simulink model "dmpwalk2014"  (R2018b)
settings: Solver=VariableStepAuto  StartTime=0.0  StopTime=100  RelTol=1e-3
values from neighbouring files (symbols this model uses):
  arm_radius = leg_radius    (= 0.01)    [Nao_paramter.m]
  foot_height = 0.02    [Nao_paramter.m]
  foot_length = 0.1    [Nao_paramter.m]
  foot_mass = 0.17184    [Nao_paramter.m]
  foot_width = 0.05    [Nao_paramter.m]
  ground_height = 0.0025    [Nao_paramter.m]
  ground_length = 5    [Nao_paramter.m]
  ground_width = 2    [Nao_paramter.m]
  hand_mass = 0.18533    [Nao_paramter.m]
  head_mass = 0.60533    [Nao_paramter.m]
  hip_mass = 0.14053    [Nao_paramter.m]
  hip_off_Y = 0.05    [Nao_paramter.m]
  hip_off_Z = 0.085    [Nao_paramter.m]
  leg_radius = 0.01    [Nao_paramter.m]
  lowerarm_length = 0.05595    [Nao_paramter.m]
  lowerarm_mass = 0.07761    [Nao_paramter.m]
  neck_length = 0.03    [Nao_paramter.m]
  neck_mass = 0.07842    [Nao_paramter.m]
  neck_off_Z = 0.1265    [Nao_paramter.m]
  shoulder_mass = 0.09304    [Nao_paramter.m]
  thigh_mass = 0.38968    [Nao_paramter.m]
  tibia_mass = 0.30142    [Nao_paramter.m]
  torso_height = foot_height + tibia_length + thigh_length + 0.5*hip_off_Z    (= 0.2654)    [Nao_paramter.m]
  torso_mass = 1.0496    [Nao_paramter.m]
  upperarm_length = 0.105    [Nao_paramter.m]
  upperarm_mass = 0.15777    [Nao_paramter.m]
undefined symbols (not defined in the file or in its folder): sigbuilder_block, X, Y, Z
libraries: sm_lib x87, nesl_utility x15, Contact_Forces_Lib x10
(part 5 of 5)

== stateflow chart dmpwalk2014/motion planning2 ==
  state startStep
    entry:
    tau = 1;
    sDStart = tau*2.04;
    kStartMax = sDStart*100+1;
    [hPil,hPir,kBel,kBer,aPil,aPir,hRol,hRor,aRol,aRor,hYal,hYar] = motionStart(tau);
    state outStart
      entry:
      k = k+1;
      hipRollR = hRor(k);
      hipRollL = hRol(k);
      hipPitchR = hPir(k);
      hipPitchL = hPil(k);
      hipYawR = hYar(k);
      hipYawL = hYal(k);
      kneeBendR = kBer(k);
      kneeBendL = kBel(k);
      ankleRollR = aRor(k);
      ankleRollL = aRol(k);
      anklePitchR = aPir(k);
      anklePitchL = aPil(k);
    (default) -> outStart : {k=0;}
    outStart -> outStart : after(0.01,sec)[k < kStartMax]
  state stepLeft
    entry:
    sDStraight = tau*2.05 ;
    kStraightMax = sDStraight*100+1;
    [hPil,hPir,kBel,kBer,aPil,aPir,hRol,hRor,aRol,aRor,hYal,hYar] = motionStraight(tau,countStraight,motionStartFinal,motionStraightFinal);
    state outLeft
      entry:
      k = k+1;
      hipRollR = hRor(k);
      hipRollL = hRol(k);
      hipPitchR = hPir(k);
      hipPitchL = hPil(k);
      hipYawR = hYar(k);
      hipYawL = hYal(k);
      kneeBendR = kBer(k);
      kneeBendL = kBel(k);
      ankleRollR = aRor(k);
      ankleRollL = aRol(k);
      anklePitchR = aPir(k);
      anklePitchL = aPil(k);
    (default) -> outLeft : {k=0;}
    outLeft -> outLeft : after(0.01,sec)[k < kStraightMax]
  state stepEnd
    entry:
    sDEnd = tau*2.28 ;
    kEndMax = sDEnd*100+1
    [hPil,hPir,kBel,kBer,aPil,aPir,hRol,hRor,aRol,aRor,hYal,hYar] = motionEnd(tau,countEnd,motionStraightFinal,motionEndFinal);
    state outEnd
      entry:
      k = k+1;
      hipRollR = hRor(k);
      hipRollL = hRol(k);
      hipPitchR = hPir(k);
      hipPitchL = hPil(k);
      hipYawR = hYar(k);
      hipYawL = hYal(k);
      kneeBendR = kBer(k);
      kneeBendL = kBel(k);
      ankleRollR = aRor(k);
      ankleRollL = aRol(k);
      anklePitchR = aPir(k);
      anklePitchL = aPil(k);
    (default) -> outEnd : {k=0;}
    outEnd -> outEnd : after(0.01,sec)[k < kEndMax]
  state stepSideR1
    entry:
    sDSideL = tau*2.13;
    kSideLMax = sDSideL*100+1
    [hPil,hPir,kBel,kBer,aPil,aPir,hRol,hRor,aRol,aRor,hYal,hYar] = motionSideLeft(tau,countSide,motionEndFinal,motionSideFinal);
    state outSideR
      entry:
      k = k+1;
      hipRollR = hRor(k);
      hipRollL = hRol(k);
      hipPitchR = hPir(k);
      hipPitchL = hPil(k);
      hipYawR = hYar(k);
      hipYawL = hYal(k);
      kneeBendR = kBer(k);
      kneeBendL = kBel(k);
      ankleRollR = aRor(k);
      ankleRollL = aRol(k);
      anklePitchR = aPir(k);
      anklePitchL = aPil(k);
    (default) -> outSideR : {k=0;}
    outSideR -> outSideR : after(0.01,sec)[k < kSideLMax]
  state stepSideR
    entry:
    sDSideR = tau*2.13;
    kSideRMax = sDSideR*100+1
    [hPil,hPir,kBel,kBer,aPil,aPir,hRol,hRor,aRol,aRor,hYal,hYar] = motionSideRight(tau,countSide,motionEndFinal,motionSideFinal);
    state outSideL
      entry:
      k = k+1;
      hipRollR = hRor(k);
      hipRollL = hRol(k);
      hipPitchR = hPir(k);
      hipPitchL = hPil(k);
      hipYawR = hYar(k);
      hipYawL = hYal(k);
      kneeBendR = kBer(k);
      kneeBendL = kBel(k);
      ankleRollR = aRor(k);
      ankleRollL = aRol(k);
      anklePitchR = aPir(k);
      anklePitchL = aPil(k);
    (default) -> outSideL : {k=0;}
    outSideL -> outSideL : after(0.01,sec)[k < kSideRMax]
  state stepKick
    entry:
    sDKick = tau*2.8 ;
    kKickMax = sDKick*100+1
    [hPil,hPir,kBel,kBer,aPil,aPir,hRol,hRor,aRol,aRor,hYal,hYar] = motionKick(tau,countKick,motionSideFinal,motionKickFinal);
    state outStraight
      entry:
      k = k+1;
      hipRollR = -hRor(k);
      hipRollL = -hRol(k);
      hipPitchR = hPir(k);
      hipPitchL = hPil(k);
      hipYawR = hYar(k);
      hipYawL = hYal(k);
      kneeBendR = kBer(k);
      kneeBendL = kBel(k);
      ankleRollR = -aRor(k);
      ankleRollL = -aRol(k);
      anklePitchR = aPir(k);
      anklePitchL = aPil(k);
    (default) -> outStraight : {k=0;}
    outStraight -> outStraight : after(0.01,sec)[k < kKickMax]
  state stop
    entry:
    stop = 1;
    stopWalking(stop);
    state stopWalking(in) [function]
  (default) -> startStep
  startStep -> stepLeft : after(sDStart,sec){nStraight = 10; countStraight=1;motionStraightFinal = zeros(10,1);motionStraighFinal = zeros(10,1);motionStartFinal = [hPil(k);hPir(k);kBel(k);kBer(k);aPil(k);aPir(k);hRol(k);hRor(k);aRol(k);aRor(k)]; tau = 1;}
  stepLeft -> (junction 880) : after(sDStraight,sec){nStraight = nStraight - 1;motionStraightFinal = [hPil(k);hPir(k);kBel(k);kBer(k);aPil(k);aPir(k);hRol(k);hRor(k);aRol(k);aRor(k)];}
  (junction 880) -> stepEnd [order 2] : [nStraight < 0]{nEnd = 1; countEnd = 1; motionEndFinal = zeros(10,1);tau=1}
  (junction 880) -> stepLeft [order 1] : [nStraight > 0]{countStraight = countStraight+1;}
  stepEnd -> (junction 914) : after(sDEnd,sec){nSide = 20; countSide = 1; motionEndFinal = [hPil(k);hPir(k);kBel(k);kBer(k);aPil(k);aPir(k);hRol(k);hRor(k);aRol(k);aRor(k)]; motionSideFinal = zeros(10,1); LR = 1; tau = 1}
  (junction 914) -> stepSideR1 [order 1] : [LR == 1]
  (junction 914) -> stepSideR [order 2] : [LR == 0]
  (junction 918) -> stepSideR [order 1] : [nSide > 0]{countSide = countSide+1;}
  (junction 918) -> stepSideR1 [order 2] : [nSide > 0]{countSide = countSide+1;}
  stepSideR1 -> (junction 918) : after(sDSideL,sec){nSide = nSide-1;motionSideFinal = [hPil(k);hPir(k);kBel(k);kBer(k);aPil(k);aPir(k);hRol(k);hRor(k);aRol(k);aRor(k)]}
  stepSideR -> (junction 918) : after(sDSideR,sec){nSide = nSide-1;motionSideFinal = [hPil(k);hPir(k);kBel(k);kBer(k);aPil(k);aPir(k);hRol(k);hRor(k);aRol(k);aRor(k)]}
  (junction 918) -> stepKick [order 3] : [after(nSide <= 0,sec]){nKick = 1; countKick = 1; mtionKickFinal = zeros(10,1);}
  (junction 688) -> stepKick [order 1] : [nKick > 0]{countKick = countKick+1;}
  stepKick -> (junction 688) : after(sDKick,sec){nKick = nKick-1; motionKickFinal = [hPil(k);hPir(k);kBel(k);kBer(k);aPil(k);aPir(k);hRol(k);hRor(k);aRol(k);aRor(k)];}
  (junction 688) -> stop [order 2] : [nKick <= 0]
  data: hPl function_output; hPr function_output; kBl function_output; kBr function_output; aPl function_output; aPr function_output; hRl function_output; tScale function_input; hRr function_output; aRl function_output; aRr function_output; hYl function_output; hYr function_output; hPl function_output; hPr function_output; kBl function_output; kBr function_output; aPl function_output; aPr function_output; hRl function_output; tScale function_input; count function_input; hRr function_output; aRl function_output; aRr function_output; hYl function_output; hYr function_output; ygStart function_input; ygStraight function_input; hPl function_output; hPr function_output; kBl function_output; kBr function_output; aPl function_output; aPr function_output; hRl function_output; tScale function_input; count function_input; ygStraight function_input; hRr function_output; aRl function_output; aRr function_output; hYl function_output; hYr function_output; ygEnd function_input; hPl function_output; hPr function_output; kBl function_output; kBr function_output; aPl function_output; aPr function_output; hRl function_output; tScale function_input; count function_input; ygEnd function_input; hRr function_output; aRl function_output; aRr function_output; hYl function_output; hYr function_output; ygSideLeft function_input; hPl function_output; hPr function_output; kBl function_output; kBr function_output; aPl function_output; aPr function_output; hRl function_output; tScale function_input; count function_input; ygEnd function_input; ygSideRight function_input; hRr function_output; aRl function_output; aRr function_output; hYl function_output; hYr function_output; hPl function_output; hPr function_output; kBl function_output; kBr function_output; aPl function_output; aPr function_output; hRl function_output; tScale function_input; count function_input; ygSide function_input; hRr function_output; aRl function_output; aRr function_output; hYl function_output; hYr function_output; ygKick function_input; in function_input double size=1; hipRollL output; hipRollR output; hipPitchL output; hipPitchR output; hipYawL output; hipYawR output; kneeBendL output; kneeBendR output; rp input; lp input; k local; ankleRollL output; ankleRollR output; anklePitchL output; anklePitchR output; aPil local size=[1 2000]; aPir local size=[1 2000]; aRol local size=[1 2000]; aRor local size=[1 2000]; hPil local size=[1 2000]; hPir local size=[1 2000]; hRol local size=[1 2000]; hRor local size=[1 2000]; hYal local size=[1 2000]; hYar local size=[1 2000]; kBel local size=[1 2000]; kBer local size=[1 2000]; tau local; sDStart local; kStartMax local; nStraight local; motionStartFinal local; countSide local; motionSideFinal local double size=[10 1]; nSide local; countEnd local; kEndMax local; motionEndFinal local; nEnd local; sDEnd local; stop local; sDKick local; nKick local; motionKickFinal local; kKickMax local; countKick local; LR local; kSideLMax local; kSideRMax local; sDSideL local; sDSideR local; countStraight local; motionStraighFinal local; sDStraight local; kStraightMax local; motionStraightFinal local; mtionKickFinal local
  function [hPl,hPr,kBl,kBr,aPl,aPr,hRl,hRr,aRl,aRr,hYl,hYr] = motionStart(tScale):
    | function [hPl,hPr,kBl,kBr,aPl,aPr,hRl,hRr,aRl,aRr,hYl,hYr] = motionStart(tScale)
    | 
    | 
    | w = load ('wStart.mat');
    | p = load ('primiBegH.mat');
    | 
    | dt = 0.01;
    | N_dmp = 10;     % number of dmps, number of curves to be imitated 
    | N_bf = 100;     % number of basic activation function
    | weights = zeros(N_dmp,N_bf);
    | ay = 25;        % ay & by: constants of the second order system
    | by = ay/4;
    | t = 0:dt:dt*(size(p.primiBegH,2)-1);
    | t1 = 0:dt:tScale*t(end); 
    | anglesIm1 = zeros(10,length(t1));
    | ax = 1;
    | %%
    | for j = 1:N_dmp
    |     
    |     y0 = p.primiBegH(j,1);
    |     yg = p.primiBegH(j,end);
    |     x1 = exp(-ax/tScale*t1);
    |     des_c1 = linspace(0,max(t1),N_bf);    % point in time where to put the activation function
    |     c1 = exp(-ax/tScale*des_c1);             % point in x where to put the activation function
    |     h1 = N_bf^1.5*ones(1,N_bf)./c1;       % variance of each activation function, trial and error
    | 
    |     psi1 = zeros(N_bf,length(x1));
    |         for k = 1:N_bf
    |             for l = 1:length(x1)
    |                 psi1(k,l) = exp(-h1(k)*(x1(l)-c1(k))^2);
    |             end
    |         end    
    |         
    |     % Forcing term
    |     wpsi1 = w.wStart(j,:)*psi1;
    |     f1 = wpsi1./(sum(psi1)).*x1*(yg-y0);
    |     
    |     % Reproducing
    |     ddyIm = zeros(1,length(t1));
    |     dyIm = zeros(1,length(t1));
    |     yIm = zeros(1,length(t1));
    |     yIm(1) = y0;
    |     
    |     for k = 2:length(t1)
    |         ddyIm(k-1) = 1/tau^2*(ay*(by*(yg-yIm(k-1))-tau*dyIm(k-1))+f1(k-1));
    |         dyIm(k) = dyIm(k-1)+ddyIm(k-1)*dt;
    |         yIm(k) = yIm(k-1)+dyIm(k-1)*dt;
    |     end
    |     
    |     anglesIm1(j,:) = yIm;
    | end
    | 
    | 
    | 
    | 
    | 
    | hPl = anglesIm1(1,:);
    | hPr = anglesIm1(2,:);
    | kBl = anglesIm1(3,:);
    | kBr = anglesIm1(4,:);
    | aPl = anglesIm1(5,:);
    | aPr = anglesIm1(6,:);
    | hRl = -anglesIm1(7,:);
    | hRr = -anglesIm1(8,:);
    | aRl = -anglesIm1(9,:);
    | aRr = -anglesIm1(10,:);
    | hYl = zeros(1,size(anglesIm1,2));   
    | hYr = zeros(1,size(anglesIm1,2));
  function [hPl,hPr,kBl,kBr,aPl,aPr,hRl,hRr,aRl,aRr,hYl,hYr] = motionStraight(tScale,count,ygStart,ygStraight):
    | function [hPl,hPr,kBl,kBr,aPl,aPr,hRl,hRr,aRl,aRr,hYl,hYr] = motionStraight(tScale,count,ygStart,ygStraight)
    | 
    | 
    | w = load ('wStraight.mat');
    | p = load ('primiStrW.mat');
    | 
    | dt = 0.01;
    | N_dmp = 10;     % number of dmps, number of curves to be imitated 
    | N_bf = 100;     % number of basic activation function
    | weights = zeros(N_dmp,N_bf);
    | ay = 25;        % ay & by: constants of the second order system
    | by = ay/4;
    | t = 0:dt:dt*(size(p.primiStrW,2)-1);
    | t1 = 0:dt:tScale*t(end);
    | anglesIm1 = zeros(10,length(t1));
    | ax = 1;
    | %%
    | for j = 1:N_dmp
    |     
    |     y0 = p.primiStrW(j,1);
    |     yg = p.primiStrW(j,end);
    |     x1 = exp(-ax/tScale*t1);
    |     des_c1 = linspace(0,max(t1),N_bf);    % point in time where to put the activation function
    |     c1 = exp(-ax/tScale*des_c1);             % point in x where to put the activation function
    |     h1 = N_bf^1.5*ones(1,N_bf)./c1;       % variance of each activation function, trial and error
    | 
    |     psi1 = zeros(N_bf,length(x1));
    |         for k = 1:N_bf
    |             for l = 1:length(x1)
    |                 psi1(k,l) = exp(-h1(k)*(x1(l)-c1(k))^2);
    |             end
    |         end    
    |         
    |     % Forcing term
    |     wpsi1 = w.wStraight(j,:)*psi1;
    |     f1 = wpsi1./(sum(psi1)).*x1*(yg-y0);
    |     
    |     % Reproducing
    |     ddyIm = zeros(1,length(t1));
    |     dyIm = zeros(1,length(t1));
    |     yIm = zeros(1,length(t1));
    |     
    |     if count == 1
    |         yIm(1) = ygStart(j,1);
    |     else
    |         yIm(1) = ygStraight(j,1);
    |     end
    | 
    |     
    |     
    |     for k = 2:length(t1)
    |         ddyIm(k-1) = 1/tau^2*(ay*(by*(yg-yIm(k-1))-tau*dyIm(k-1))+f1(k-1));
    |         dyIm(k) = dyIm(k-1)+ddyIm(k-1)*dt;
    |         yIm(k) = yIm(k-1)+dyIm(k-1)*dt;  
    |     end
    |     
    |     anglesIm1(j,:) = yIm;
    | end
    | 
    | 
    | hPl = anglesIm1(1,:);
    | hPr = anglesIm1(2,:);
    | kBl = anglesIm1(3,:);
    | kBr = anglesIm1(4,:);
    | aPl = anglesIm1(5,:);
    | aPr = anglesIm1(6,:);
    | hRl = -anglesIm1(7,:);
    | hRr = -anglesIm1(8,:);
    | aRl = -anglesIm1(9,:);
    | aRr = -anglesIm1(10,:);
    | hYl = zeros(1,size(anglesIm1,2));   
    | hYr = zeros(1,size(anglesIm1,2));
  function [hPl,hPr,kBl,kBr,aPl,aPr,hRl,hRr,aRl,aRr,hYl,hYr] = motionEnd(tScale,count,ygStraight,ygEnd):
    | function [hPl,hPr,kBl,kBr,aPl,aPr,hRl,hRr,aRl,aRr,hYl,hYr] = motionEnd(tScale,count,ygStraight,ygEnd)
    | 
    | 
    | w = load ('wEnd.mat');
    | p = load ('primiEndH.mat');
    | 
    | dt = 0.01;
    | N_dmp = 10;     % number of dmps, number of curves to be imitated 
    | N_bf = 100;     % number of basic activation function
    | weights = zeros(N_dmp,N_bf);
    | ay = 25;        % ay & by: constants of the second order system
    | by = ay/4;
    | t = 0:dt:dt*(size(p.primiEndH,2)-1);
    | t1 = 0:dt:tScale*t(end);
    | anglesIm1 = zeros(10,length(t1));
    | ax = 1;
    | %%
    | for j = 1:N_dmp
    |     
    |     y0 = p.primiEndH(j,1);
    |     yg = p.primiEndH(j,end);
    |     x1 = exp(-ax/tScale*t1);
    |     des_c1 = linspace(0,max(t1),N_bf);    % point in time where to put the activation function
    |     c1 = exp(-ax/tScale*des_c1);             % point in x where to put the activation function
    |     h1 = N_bf^1.5*ones(1,N_bf)./c1;       % variance of each activation function, trial and error
    | 
    |     psi1 = zeros(N_bf,length(x1));
    |         for k = 1:N_bf
    |             for l = 1:length(x1)
    |                 psi1(k,l) = exp(-h1(k)*(x1(l)-c1(k))^2);
    |             end
    |         end    
    |         
    |     % Forcing term
    |     wpsi1 = w.wEnd(j,:)*psi1;
    |     f1 = wpsi1./(sum(psi1)).*x1*(yg-y0);
    |     
    |     % Reproducing
    |     ddyIm = zeros(1,length(t1));
    |     dyIm = zeros(1,length(t1));
    |     yIm = zeros(1,length(t1));
    |     
    |     if count == 1
    |         yIm(1) = ygStraight(j,1);
    |     else
    |         yIm(1) = ygEnd(j,1);
    |     end
    | 
    |     
    |     
    |     for k = 2:length(t1)
    |         ddyIm(k-1) = 1/tau^2*(ay*(by*(yg-yIm(k-1))-tau*dyIm(k-1))+f1(k-1));
    |         dyIm(k) = dyIm(k-1)+ddyIm(k-1)*dt;
    |         yIm(k) = yIm(k-1)+dyIm(k-1)*dt;  
    |     end
    |     
    |     anglesIm1(j,:) = yIm;
    | end
    | 
    | 
    | hPl = anglesIm1(1,:);
    | hPr = anglesIm1(2,:);
    | kBl = anglesIm1(3,:);
    | kBr = anglesIm1(4,:);
    | aPl = anglesIm1(5,:);
    | aPr = anglesIm1(6,:);
    | hRl = -anglesIm1(7,:);
    | hRr = -anglesIm1(8,:);
    | aRl = -anglesIm1(9,:);
    | aRr = -anglesIm1(10,:);
    | hYl = zeros(1,size(anglesIm1,2));   
    | hYr = zeros(1,size(anglesIm1,2));
  function [hPl,hPr,kBl,kBr,aPl,aPr,hRl,hRr,aRl,aRr,hYl,hYr] = motionSideLeft(tScale,count,ygEnd,ygSideLeft):
    | function [hPl,hPr,kBl,kBr,aPl,aPr,hRl,hRr,aRl,aRr,hYl,hYr] = motionSideLeft(tScale,count,ygEnd,ygSideLeft)
    | 
    | 
    | w = load ('wSideL.mat');
    | p = load ('primiSideWL.mat');
    | 
    | dt = 0.01;
    | N_dmp = 10;     % number of dmps, number of curves to be imitated 
    | N_bf = 100;     % number of basic activation function
    | weights = zeros(N_dmp,N_bf);
    | ay = 25;        % ay & by: constants of the second order system
    | by = ay/4;
    | t = 0:dt:dt*(size(p.primiSideWL,2)-1);
    | t1 = 0:dt:tScale*t(end);
    | anglesIm1 = zeros(10,length(t1));
    | ax = 1;
    | %%
    | for j = 1:N_dmp
    |    
    |     y0 = p.primiSideWL(j,1);
    |     yg = p.primiSideWL(j,end);
    | 
    | 
    |     x1 = exp(-ax/tScale*t1);
    |     des_c1 = linspace(0,max(t1),N_bf);    % point in time where to put the activation function
    |     c1 = exp(-ax/tScale*des_c1);             % point in x where to put the activation function
    |     h1 = N_bf^1.5*ones(1,N_bf)./c1;       % variance of each activation function, trial and error
    | 
    |     psi1 = zeros(N_bf,length(x1));
    |         for k = 1:N_bf
    |             for l = 1:length(x1)
    |                 psi1(k,l) = exp(-h1(k)*(x1(l)-c1(k))^2);
    |             end
    |         end    
    |         
    |     % Forcing term
    |     
    |     wpsi1 = w.wSideL(j,:)*psi1;
    |     f1 = wpsi1./(sum(psi1)).*x1*(yg-y0);
    |     
    |     % Reproducing
    |     ddyIm = zeros(1,length(t1));
    |     dyIm = zeros(1,length(t1));
    |     yIm = zeros(1,length(t1));
    |     
    |     if count == 1
    |         yIm(1) = ygEnd(j,1);
    |     else
    |         yIm(1) = ygSideLeft(j,1);
    |     end
    | 
    |     
    |     
    |     for k = 2:length(t1)
    |         ddyIm(k-1) = 1/tau^2*(ay*(by*(yg-yIm(k-1))-tau*dyIm(k-1))+f1(k-1));
    |         dyIm(k) = dyIm(k-1)+ddyIm(k-1)*dt;
    |         yIm(k) = yIm(k-1)+dyIm(k-1)*dt;
    |     end
    |     
    |     anglesIm1(j,:) = yIm;
    | end
    | 
    | 
    | hPl = anglesIm1(1,:);
    | hPr = anglesIm1(2,:);
    | kBl = anglesIm1(3,:);
    | kBr = anglesIm1(4,:);
    | aPl = anglesIm1(5,:);
    | aPr = anglesIm1(6,:);
    | hRl = -anglesIm1(7,:);
    | hRr = -anglesIm1(8,:);
    | aRl = -anglesIm1(9,:);
    | aRr = -anglesIm1(10,:);
    | hYl = zeros(1,size(anglesIm1,2));   
    | hYr = zeros(1,size(anglesIm1,2));
  function [hPl,hPr,kBl,kBr,aPl,aPr,hRl,hRr,aRl,aRr,hYl,hYr] = motionSideRight(tScale,count,ygEnd,ygSideRight):
    | function [hPl,hPr,kBl,kBr,aPl,aPr,hRl,hRr,aRl,aRr,hYl,hYr] = motionSideRight(tScale,count,ygEnd,ygSideRight)
    | 
    | 
    | w = load ('wSideR.mat');
    | p = load ('primiSideWR.mat');
    | 
    | dt = 0.01;
    | N_dmp = 10;     % number of dmps, number of curves to be imitated 
    | N_bf = 100;     % number of basic activation function
    | weights = zeros(N_dmp,N_bf);
    | ay = 25;        % ay & by: constants of the second order system
    | by = ay/4;
    | t = 0:dt:dt*(size(p.primiSideWR,2)-1);
    | t1 = 0:dt:tScale*t(end);
    | anglesIm1 = zeros(10,length(t1));
    | ax = 1;
    | %%
    | for j = 1:N_dmp
    |    
    |     y0 = p.primiSideWR(j,1);
    |     yg = p.primiSideWR(j,end);
    | 
    | 
    |     x1 = exp(-ax/tScale*t1);
    |     des_c1 = linspace(0,max(t1),N_bf);    % point in time where to put the activation function
    |     c1 = exp(-ax/tScale*des_c1);             % point in x where to put the activation function
    |     h1 = N_bf^1.5*ones(1,N_bf)./c1;       % variance of each activation function, trial and error
    | 
    |     psi1 = zeros(N_bf,length(x1));
    |         for k = 1:N_bf
    |             for l = 1:length(x1)
    |                 psi1(k,l) = exp(-h1(k)*(x1(l)-c1(k))^2);
    |             end
    |         end    
    |         
    |     % Forcing term
    |     
    |     wpsi1 = w.wSideR(j,:)*psi1;
    |     f1 = wpsi1./(sum(psi1)).*x1*(yg-y0);
    |     
    |     % Reproducing
    |     ddyIm = zeros(1,length(t1));
    |     dyIm = zeros(1,length(t1));
    |     yIm = zeros(1,length(t1));
    |     
    |     if count == 1
    |         yIm(1) = ygEnd(j,1);
    |     else
    |         yIm(1) = ygSideRight(j,1);
    |     end
    | 
    |     
    |     
    |     for k = 2:length(t1)
    |         ddyIm(k-1) = 1/tau^2*(ay*(by*(yg-yIm(k-1))-tau*dyIm(k-1))+f1(k-1));
    |         dyIm(k) = dyIm(k-1)+ddyIm(k-1)*dt;
    |         yIm(k) = yIm(k-1)+dyIm(k-1)*dt;  
    |     end
    |     
    |     anglesIm1(j,:) = yIm;
    | end
    | 
    | 
    | hPl = anglesIm1(1,:);
    | hPr = anglesIm1(2,:);
    | kBl = anglesIm1(3,:);
    | kBr = anglesIm1(4,:);
    | aPl = anglesIm1(5,:);
    | aPr = anglesIm1(6,:);
    | hRl = -anglesIm1(7,:);
    | hRr = -anglesIm1(8,:);
    | aRl = -anglesIm1(9,:);
    | aRr = -anglesIm1(10,:);
    | hYl = zeros(1,size(anglesIm1,2));   
    | hYr = zeros(1,size(anglesIm1,2));
  function [hPl,hPr,kBl,kBr,aPl,aPr,hRl,hRr,aRl,aRr,hYl,hYr] = motionKick(tScale,count,ygSide,ygKick):
    | function [hPl,hPr,kBl,kBr,aPl,aPr,hRl,hRr,aRl,aRr,hYl,hYr] = motionKick(tScale,count,ygSide,ygKick)
    | 
    | 
    | w = load ('wKick.mat');
    | p = load ('primiKick.mat');
    | 
    | dt = 0.01;
    | N_dmp = 10;     % number of dmps, number of curves to be imitated 
    | N_bf = 100;     % number of basic activation function
    | weights = zeros(N_dmp,N_bf);
    | ay = 25;        % ay & by: constants of the second order system
    | by = ay/4;
    | t = 0:dt:dt*(size(p.primiKick,2)-1);
    | t1 = 0:dt:tScale*t(end);
    | anglesIm1 = zeros(10,length(t1));
    | ax = 1;
    | %%
    | for j = 1:N_dmp
    |     
    |     y0 = p.primiKick(j,1);
    |     yg = p.primiKick(j,end);
    |     x1 = exp(-ax/tScale*t1);
    |     des_c1 = linspace(0,max(t1),N_bf);    % point in time where to put the activation function
    |     c1 = exp(-ax/tScale*des_c1);             % point in x where to put the activation function
    |     h1 = N_bf^1.5*ones(1,N_bf)./c1;       % variance of each activation function, trial and error
    | 
    |     psi1 = zeros(N_bf,length(x1));
    |         for k = 1:N_bf
    |             for l = 1:length(x1)
    |                 psi1(k,l) = exp(-h1(k)*(x1(l)-c1(k))^2);
    |             end
    |         end    
    |         
    |     % Forcing term
    |     wpsi1 = w.wKick(j,:)*psi1;
    |     f1 = wpsi1./(sum(psi1)).*x1*(yg-y0);
    |     
    |     % Reproducing
    |     ddyIm = zeros(1,length(t1));
    |     dyIm = zeros(1,length(t1));
    |     yIm = zeros(1,length(t1));
    |     
    |     if count == 1
    |         yIm(1) = ygSide(j,1);
    |     else
    |         yIm(1) = ygKick(j,1);
    |     end
    | 
    |     
    |     
    |     for k = 2:length(t1)
    |         ddyIm(k-1) = 1/tau^2*(ay*(by*(yg-yIm(k-1))-tau*dyIm(k-1))+f1(k-1));
    |         dyIm(k) = dyIm(k-1)+ddyIm(k-1)*dt;
    |         yIm(k) = yIm(k-1)+dyIm(k-1)*dt;
    |     end
    |     
    |     anglesIm1(j,:) = yIm;
    | end
    | 
    | 
    | hPl = anglesIm1(1,:);
    | hPr = anglesIm1(2,:);
    | kBl = anglesIm1(3,:);
    | kBr = anglesIm1(4,:);
    | aPl = anglesIm1(5,:);
    | aPr = anglesIm1(6,:);
    | hRl = anglesIm1(7,:);
    | hRr = anglesIm1(8,:);
    | aRl = anglesIm1(9,:);
    | aRr = anglesIm1(10,:);
    | hYl = zeros(1,size(anglesIm1,2));   
    | hYr = zeros(1,size(anglesIm1,2));
